simulink library "BechamoNasaOpenModels"  (R2024b)
settings: Solver=VariableStepAuto  StartTime=0.0  StopTime=10.0  RelTol=1e-3
values from neighbouring files (symbols this model uses):
  Cl_aileron_wing_1 = Cl_mat.Claileron_wing.axes1.value    [setupMavrik.m]
  Cl_aileron_wing_2 = Cl_mat.Claileron_wing.axes2.value    [setupMavrik.m]
  Cl_aileron_wing_3 = Cl_mat.Claileron_wing.axes3.value    [setupMavrik.m]
  Cl_aileron_wing_val = Cl_mat.Claileron_wing.value    [setupMavrik.m]
  Cl_elevator_tail_1 = Cl_mat.Clelevator_tail.axes1.value    [setupMavrik.m]
  Cl_elevator_tail_2 = Cl_mat.Clelevator_tail.axes2.value    [setupMavrik.m]
  Cl_elevator_tail_3 = Cl_mat.Clelevator_tail.axes3.value    [setupMavrik.m]
  Cl_elevator_tail_val = Cl_mat.Clelevator_tail.value    [setupMavrik.m]
  Cl_flap_wing_1 = Cl_mat.Clflap_wing.axes1.value    [setupMavrik.m]
  Cl_flap_wing_2 = Cl_mat.Clflap_wing.axes2.value    [setupMavrik.m]
  Cl_flap_wing_3 = Cl_mat.Clflap_wing.axes3.value    [setupMavrik.m]
  Cl_flap_wing_val = Cl_mat.Clflap_wing.value    [setupMavrik.m]
  Cl_hover_fuse_1 = Cl_mat.Clhover_fuse.axes1.value    [setupMavrik.m]
  Cl_hover_fuse_2 = Cl_mat.Clhover_fuse.axes2.value    [setupMavrik.m]
  Cl_hover_fuse_3 = Cl_mat.Clhover_fuse.axes3.value    [setupMavrik.m]
  Cl_hover_fuse_val = Cl_mat.Clhover_fuse.value    [setupMavrik.m]
  Cl_rudder_tail_1 = Cl_mat.Clrudder_tail.axes1.value    [setupMavrik.m]
  Cl_rudder_tail_2 = Cl_mat.Clrudder_tail.axes2.value    [setupMavrik.m]
  Cl_rudder_tail_3 = Cl_mat.Clrudder_tail.axes3.value    [setupMavrik.m]
  Cl_rudder_tail_val = Cl_mat.Clrudder_tail.value    [setupMavrik.m]
  Cl_tail_1 = Cl_mat.Cltail.axes1.value    [setupMavrik.m]
  Cl_tail_2 = Cl_mat.Cltail.axes2.value    [setupMavrik.m]
  Cl_tail_3 = Cl_mat.Cltail.axes3.value    [setupMavrik.m]
  Cl_tail_damp_p_1 = Cl_mat.Cltail_damp_p.axes1.value    [setupMavrik.m]
  Cl_tail_damp_p_2 = Cl_mat.Cltail_damp_p.axes2.value    [setupMavrik.m]
  Cl_tail_damp_p_3 = Cl_mat.Cltail_damp_p.axes3.value    [setupMavrik.m]
  Cl_tail_damp_p_val = Cl_mat.Cltail_damp_p.value    [setupMavrik.m]
  Cl_tail_damp_q_1 = Cl_mat.Cltail_damp_q.axes1.value    [setupMavrik.m]
  Cl_tail_damp_q_2 = Cl_mat.Cltail_damp_q.axes2.value    [setupMavrik.m]
  Cl_tail_damp_q_3 = Cl_mat.Cltail_damp_q.axes3.value    [setupMavrik.m]
  Cl_tail_damp_q_val = Cl_mat.Cltail_damp_q.value    [setupMavrik.m]
  Cl_tail_damp_r_1 = Cl_mat.Cltail_damp_r.axes1.value    [setupMavrik.m]
  Cl_tail_damp_r_2 = Cl_mat.Cltail_damp_r.axes2.value    [setupMavrik.m]
  Cl_tail_damp_r_3 = Cl_mat.Cltail_damp_r.axes3.value    [setupMavrik.m]
  Cl_tail_damp_r_val = Cl_mat.Cltail_damp_r.value    [setupMavrik.m]
  Cl_tail_val = Cl_mat.Cltail.value    [setupMavrik.m]
  Cl_wing_1 = Cl_mat.Clwing.axes1.value    [setupMavrik.m]
  Cl_wing_2 = Cl_mat.Clwing.axes2.value    [setupMavrik.m]
  Cl_wing_3 = Cl_mat.Clwing.axes3.value    [setupMavrik.m]
  Cl_wing_damp_p_1 = Cl_mat.Clwing_damp_p.axes1.value    [setupMavrik.m]
  Cl_wing_damp_p_2 = Cl_mat.Clwing_damp_p.axes2.value    [setupMavrik.m]
  Cl_wing_damp_p_3 = Cl_mat.Clwing_damp_p.axes3.value    [setupMavrik.m]
  Cl_wing_damp_p_val = Cl_mat.Clwing_damp_p.value    [setupMavrik.m]
  Cl_wing_damp_q_1 = Cl_mat.Clwing_damp_q.axes1.value    [setupMavrik.m]
  Cl_wing_damp_q_2 = Cl_mat.Clwing_damp_q.axes2.value    [setupMavrik.m]
  Cl_wing_damp_q_3 = Cl_mat.Clwing_damp_q.axes3.value    [setupMavrik.m]
  Cl_wing_damp_q_val = Cl_mat.Clwing_damp_q.value    [setupMavrik.m]
  Cl_wing_damp_r_1 = Cl_mat.Clwing_damp_r.axes1.value    [setupMavrik.m]
  Cl_wing_damp_r_2 = Cl_mat.Clwing_damp_r.axes2.value    [setupMavrik.m]
  Cl_wing_damp_r_3 = Cl_mat.Clwing_damp_r.axes3.value    [setupMavrik.m]
  Cl_wing_damp_r_val = Cl_mat.Clwing_damp_r.value    [setupMavrik.m]
  Cl_wing_val = Cl_mat.Clwing.value    [setupMavrik.m]
  Cm_aileron_wing_1 = Cm_mat.Cmaileron_wing.axes1.value    [setupMavrik.m]
  Cm_aileron_wing_2 = Cm_mat.Cmaileron_wing.axes2.value    [setupMavrik.m]
  Cm_aileron_wing_3 = Cm_mat.Cmaileron_wing.axes3.value    [setupMavrik.m]
  Cm_aileron_wing_val = Cm_mat.Cmaileron_wing.value    [setupMavrik.m]
  Cm_elevator_tail_1 = Cm_mat.Cmelevator_tail.axes1.value    [setupMavrik.m]
  Cm_elevator_tail_2 = Cm_mat.Cmelevator_tail.axes2.value    [setupMavrik.m]
  Cm_elevator_tail_3 = Cm_mat.Cmelevator_tail.axes3.value    [setupMavrik.m]
  Cm_elevator_tail_val = Cm_mat.Cmelevator_tail.value    [setupMavrik.m]
  Cm_flap_wing_1 = Cm_mat.Cmflap_wing.axes1.value    [setupMavrik.m]
  Cm_flap_wing_2 = Cm_mat.Cmflap_wing.axes2.value    [setupMavrik.m]
  Cm_flap_wing_3 = Cm_mat.Cmflap_wing.axes3.value    [setupMavrik.m]
  Cm_flap_wing_val = Cm_mat.Cmflap_wing.value    [setupMavrik.m]
  Cm_hover_fuse_1 = Cm_mat.Cmhover_fuse.axes1.value    [setupMavrik.m]
  Cm_hover_fuse_2 = Cm_mat.Cmhover_fuse.axes2.value    [setupMavrik.m]
  Cm_hover_fuse_3 = Cm_mat.Cmhover_fuse.axes3.value    [setupMavrik.m]
  Cm_hover_fuse_val = Cm_mat.Cmhover_fuse.value    [setupMavrik.m]
  Cm_rudder_tail_1 = Cm_mat.Cmrudder_tail.axes1.value    [setupMavrik.m]
  Cm_rudder_tail_2 = Cm_mat.Cmrudder_tail.axes2.value    [setupMavrik.m]
  Cm_rudder_tail_3 = Cm_mat.Cmrudder_tail.axes3.value    [setupMavrik.m]
  Cm_rudder_tail_val = Cm_mat.Cmrudder_tail.value    [setupMavrik.m]
  Cm_tail_1 = Cm_mat.Cmtail.axes1.value    [setupMavrik.m]
  Cm_tail_2 = Cm_mat.Cmtail.axes2.value    [setupMavrik.m]
  Cm_tail_3 = Cm_mat.Cmtail.axes3.value    [setupMavrik.m]
  Cm_tail_damp_p_1 = Cm_mat.Cmtail_damp_p.axes1.value    [setupMavrik.m]
  Cm_tail_damp_p_2 = Cm_mat.Cmtail_damp_p.axes2.value    [setupMavrik.m]
  Cm_tail_damp_p_3 = Cm_mat.Cmtail_damp_p.axes3.value    [setupMavrik.m]
  Cm_tail_damp_p_val = Cm_mat.Cmtail_damp_p.value    [setupMavrik.m]
  Cm_tail_damp_q_1 = Cm_mat.Cmtail_damp_q.axes1.value    [setupMavrik.m]
  Cm_tail_damp_q_2 = Cm_mat.Cmtail_damp_q.axes2.value    [setupMavrik.m]
  Cm_tail_damp_q_3 = Cm_mat.Cmtail_damp_q.axes3.value    [setupMavrik.m]
  Cm_tail_damp_q_val = Cm_mat.Cmtail_damp_q.value    [setupMavrik.m]
  Cm_tail_damp_r_1 = Cm_mat.Cmtail_damp_r.axes1.value    [setupMavrik.m]
  Cm_tail_damp_r_2 = Cm_mat.Cmtail_damp_r.axes2.value    [setupMavrik.m]
  Cm_tail_damp_r_3 = Cm_mat.Cmtail_damp_r.axes3.value    [setupMavrik.m]
  Cm_tail_damp_r_val = Cm_mat.Cmtail_damp_r.value    [setupMavrik.m]
  Cm_tail_val = Cm_mat.Cmtail.value    [setupMavrik.m]
  Cm_wing_1 = Cm_mat.Cmwing.axes1.value    [setupMavrik.m]
  Cm_wing_2 = Cm_mat.Cmwing.axes2.value    [setupMavrik.m]
  Cm_wing_3 = Cm_mat.Cmwing.axes3.value    [setupMavrik.m]
  Cm_wing_damp_p_1 = Cm_mat.Cmwing_damp_p.axes1.value    [setupMavrik.m]
  Cm_wing_damp_p_2 = Cm_mat.Cmwing_damp_p.axes2.value    [setupMavrik.m]
  Cm_wing_damp_p_3 = Cm_mat.Cmwing_damp_p.axes3.value    [setupMavrik.m]
  Cm_wing_damp_p_val = Cm_mat.Cmwing_damp_p.value    [setupMavrik.m]
  Cm_wing_damp_q_1 = Cm_mat.Cmwing_damp_q.axes1.value    [setupMavrik.m]
  Cm_wing_damp_q_2 = Cm_mat.Cmwing_damp_q.axes2.value    [setupMavrik.m]
  Cm_wing_damp_q_3 = Cm_mat.Cmwing_damp_q.axes3.value    [setupMavrik.m]
  Cm_wing_damp_q_val = Cm_mat.Cmwing_damp_q.value    [setupMavrik.m]
  Cm_wing_damp_r_1 = Cm_mat.Cmwing_damp_r.axes1.value    [setupMavrik.m]
  Cm_wing_damp_r_2 = Cm_mat.Cmwing_damp_r.axes2.value    [setupMavrik.m]
  Cm_wing_damp_r_3 = Cm_mat.Cmwing_damp_r.axes3.value    [setupMavrik.m]
  Cm_wing_damp_r_val = Cm_mat.Cmwing_damp_r.value    [setupMavrik.m]
  Cm_wing_val = Cm_mat.Cmwing.value    [setupMavrik.m]
  Cn_aileron_wing_1 = Cn_mat.Cnaileron_wing.axes1.value    [setupMavrik.m]
  Cn_aileron_wing_2 = Cn_mat.Cnaileron_wing.axes2.value    [setupMavrik.m]
  Cn_aileron_wing_3 = Cn_mat.Cnaileron_wing.axes3.value    [setupMavrik.m]
  Cn_aileron_wing_val = Cn_mat.Cnaileron_wing.value    [setupMavrik.m]
  Cn_elevator_tail_1 = Cn_mat.Cnelevator_tail.axes1.value    [setupMavrik.m]
  Cn_elevator_tail_2 = Cn_mat.Cnelevator_tail.axes2.value    [setupMavrik.m]
  Cn_elevator_tail_3 = Cn_mat.Cnelevator_tail.axes3.value    [setupMavrik.m]
  Cn_elevator_tail_val = Cn_mat.Cnelevator_tail.value    [setupMavrik.m]
  Cn_flap_wing_1 = Cn_mat.Cnflap_wing.axes1.value    [setupMavrik.m]
  Cn_flap_wing_2 = Cn_mat.Cnflap_wing.axes2.value    [setupMavrik.m]
  Cn_flap_wing_3 = Cn_mat.Cnflap_wing.axes3.value    [setupMavrik.m]
  Cn_flap_wing_val = Cn_mat.Cnflap_wing.value    [setupMavrik.m]
  Cn_hover_fuse_1 = Cn_mat.Cnhover_fuse.axes1.value    [setupMavrik.m]
  Cn_hover_fuse_2 = Cn_mat.Cnhover_fuse.axes2.value    [setupMavrik.m]
  Cn_hover_fuse_3 = Cn_mat.Cnhover_fuse.axes3.value    [setupMavrik.m]
  Cn_hover_fuse_val = Cn_mat.Cnhover_fuse.value    [setupMavrik.m]
  ... (+319 more)
libraries: matrix_library x15, sharedtransform x2, $bdroot x1, shared6dof x1
(part 1 of 19)
settings Model: Creator=MichaelPiedmonte  LastModifiedBy=DivyangAmin

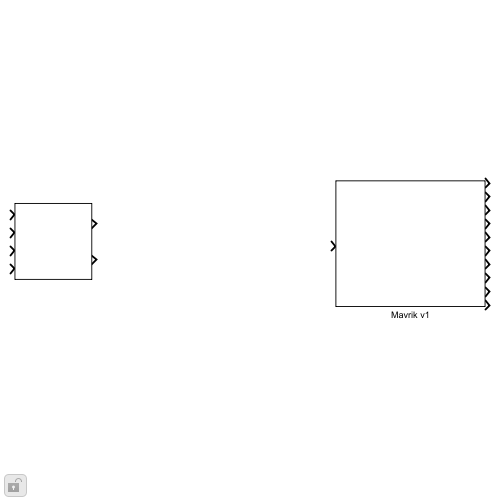
[thumbnail: Simulink's stored preview of the top-level diagram]
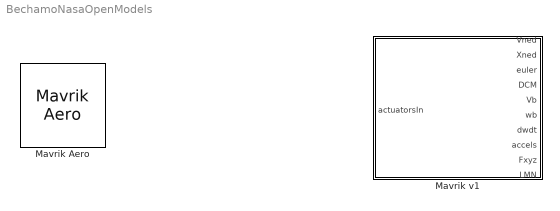
== system BechamoNasaOpenModels ==
  Mavrik Aero : $bdroot/Mavrik v1/Mavrik Aero  SystemSampleTime=-1  VariantActivationTime=update diagram  AllowFlexibleInterface=on  Latency=0  AutoFrameSizeCalculation=off
  Mavrik v1 : Subsystem  mask{uvw_init=0, pqr_init=0, euler_init=0, xyz_init=0, mass=0, inertia=0}
      mask prompts: uvw_init "uvw initial values"; pqr_init "pqr initial values"; euler_init "euler angle initial values"; xyz_init "xyz initial values"; mass "Mass (kg)"; inertia "Inertia (kg m^2)"

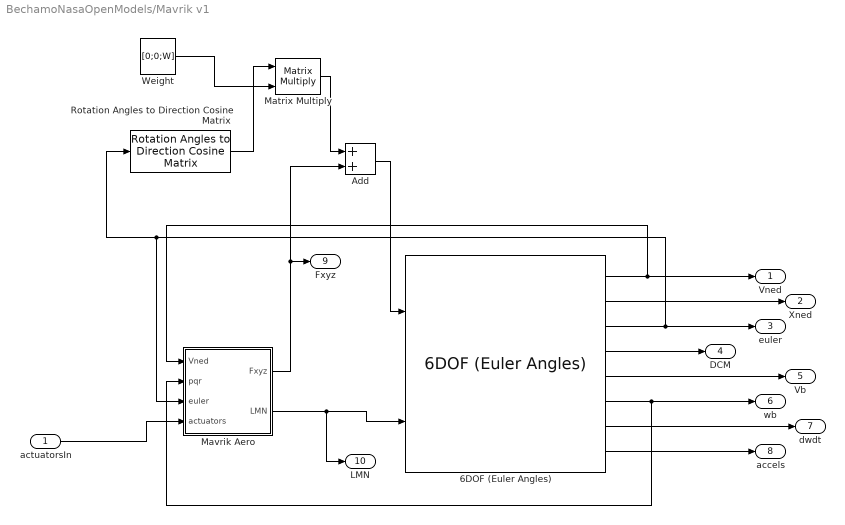
== system BechamoNasaOpenModels/Mavrik v1 ==
  actuatorsIn : Inport
  6DOF (Euler Angles) : shared6dof/6DOF (Euler Angles)  units=Metric (MKS)  mtype=Fixed  rep=Euler Angles  xme_0=xyz_init  Vm_0=uvw_init  eul_0=euler_init  pm_0=pqr_init  mass_0=mass  mass_e=0.5  mass_f=2.0  inertia=inertia  inertia_e=eye(3)  inertia_f=2*eye(3)  k_quat=1.0  vre_flag=on  abi_flag=off  aMode=0  xme_statename=''  Vm_statename=''  eul_statename=''  quat_statename=''  pm_statename=''  mass_statename=''
  Add : Sum
  Matrix Multiply : Product  Multiplication=Matrix(*)
  Mavrik Aero : Subsystem
  Rotation Angles to Direction Cosine Matrix : sharedtransform/Rotation Angles to Direction Cosine Matrix  rotationOrder=ZYX  aMode=aMode
  Weight : Constant  Value=[0;0;W]
  Vned : Outport
  Xned : Outport  Port=2
  euler : Outport  Port=3
  DCM : Outport  Port=4
  Vb : Outport  Port=5
  wb : Outport  Port=6
  dwdt : Outport  Port=7
  accels : Outport  Port=8
  Fxyz : Outport  Port=9
  LMN : Outport  Port=10
  wires:
  Mavrik Aero/2(LMN) -> LMN/1, 6DOF (Euler Angles)/2
  6DOF (Euler Angles)/6 -> Mavrik Aero/2(pqr), wb/1
  actuatorsIn/1 -> Mavrik Aero/4(actuators)
  Mavrik Aero/1(Fxyz) -> Add/2, Fxyz/1
  6DOF (Euler Angles)/1 -> Mavrik Aero/1(Vned), Vned/1
  6DOF (Euler Angles)/2 -> Xned/1
  6DOF (Euler Angles)/5 -> Vb/1
  6DOF (Euler Angles)/3 -> Rotation Angles to Direction Cosine Matrix/1, Mavrik Aero/3(euler), euler/1
  6DOF (Euler Angles)/4 -> DCM/1
  6DOF (Euler Angles)/7 -> dwdt/1
  6DOF (Euler Angles)/8 -> accels/1
  Add/1 -> 6DOF (Euler Angles)/1
  Matrix Multiply/1 -> Add/1
  Rotation Angles to Direction Cosine Matrix/1 -> Matrix Multiply/1
  Weight/1 -> Matrix Multiply/2

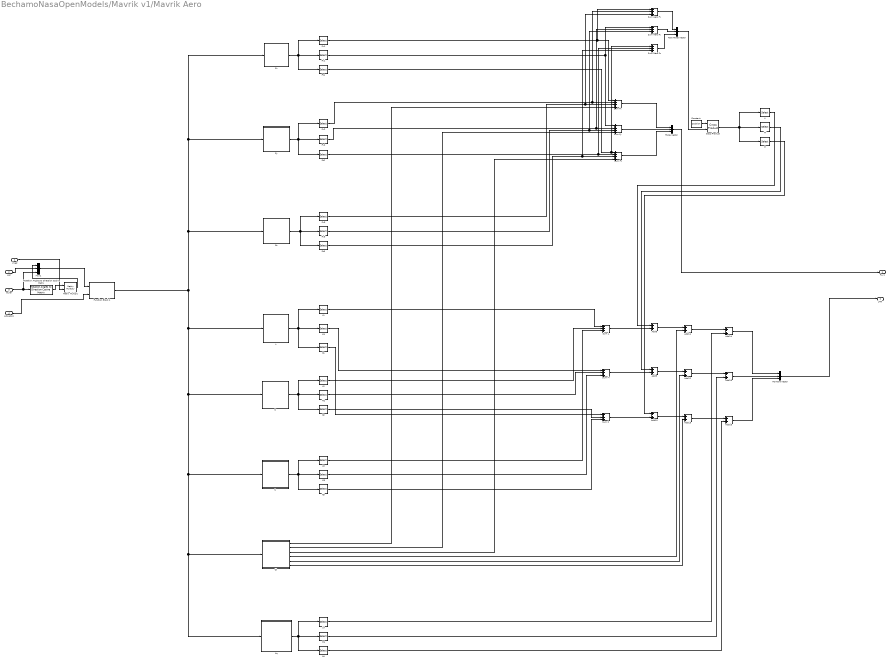
== system BechamoNasaOpenModels/Mavrik v1/Mavrik Aero ==
  Vned : Inport
  pqr : Inport  Port=2
  euler : Inport  Port=3
  actuators : Inport  Port=4
  Add{8..16} (9 alike) : Sum
  Aero Force Vector : Mux  Inputs=3
  Constant : Constant  Value=position
  Cross Product : matrix_library/Cross Product
  Ct : Subsystem
  Cx : Subsystem
  Cy : Subsystem
  Cz : Subsystem
  Force Vector : Mux  Inputs=3
  Function Block 1 : MATLAB Function  TreatAsAtomicUnit=on
  Fx1 : Selector  InputPortWidth=3  IndexOptions=Starting index (dialog)  Indices=[1]  OutputSizes=1
  Fx2 : Selector  InputPortWidth=3  IndexOptions=Starting index (dialog)  Indices=[1]  OutputSizes=1
  Fx3 : Selector  InputPortWidth=3  IndexOptions=Starting index (dialog)  Indices=[1]  OutputSizes=1
  Fy1 : Selector  InputPortWidth=3  IndexOptions=Starting index (dialog)  Indices=[2]  OutputSizes=1
  Fy2 : Selector  InputPortWidth=3  IndexOptions=Starting index (dialog)  Indices=[2]  OutputSizes=1
  Fy3 : Selector  InputPortWidth=3  IndexOptions=Starting index (dialog)  Indices=[2]  OutputSizes=1
  Fz1 : Selector  InputPortWidth=3  IndexOptions=Starting index (dialog)  Indices=[3]  OutputSizes=1
  Fz2 : Selector  InputPortWidth=3  IndexOptions=Starting index (dialog)  Indices=[3]  OutputSizes=1
  Fz3 : Selector  InputPortWidth=3  IndexOptions=Starting index (dialog)  Indices=[3]  OutputSizes=1
  Kq : Subsystem
  L : Subsystem
  L' : Selector  InputPortWidth=3  IndexOptions=Starting index (dialog)  Indices=[1]  OutputSizes=1
  L{1..4} (4 alike) : Selector  InputPortWidth=3  IndexOptions=Starting index (dialog)  Indices=[1]  OutputSizes=1
  M : Subsystem
  M' : Selector  InputPortWidth=3  IndexOptions=Starting index (dialog)  Indices=[2]  OutputSizes=1
  M{1..4} (4 alike) : Selector  InputPortWidth=3  IndexOptions=Starting index (dialog)  Indices=[2]  OutputSizes=1
  Matrix Multiply : Product  Multiplication=Matrix(*)
  Moment Vector : Mux  Inputs=3
  Mux1 : Mux  Inputs=3
  N : Subsystem
  N' : Selector  InputPortWidth=3  IndexOptions=Starting index (dialog)  Indices=[3]  OutputSizes=1
  N{1..4} (4 alike) : Selector  InputPortWidth=3  IndexOptions=Starting index (dialog)  Indices=[3]  OutputSizes=1
  Rotation Angles to Direction Cosine Matrix : sharedtransform/Rotation Angles to Direction Cosine Matrix  rotationOrder=ZYX  aMode=aMode
  Sum Aero Fx : Sum  Inputs=+++
  Sum Aero Fy : Sum  Inputs=+++
  Sum Aero Fz : Sum  Inputs=+++
  Sum Fx : Sum  Inputs=++++
  Sum Fy : Sum  Inputs=++++
  Sum Fz : Sum  Inputs=++++
  Sum L : Sum  Inputs=+++
  Sum M : Sum  Inputs=+++
  Sum N : Sum  Inputs=+++
  Fxyz : Outport
  LMN : Outport  Port=2
  wires:
  Fz1/1 -> Sum Aero Fz/1, Sum Fz/1
  Function Block 1/1(y) -> Cz/1(u), Cx/1(u), Cy/1(u), L/1(u), Kq/1(u), Ct/1(u19), N/1(u), M/1(u)
  Ct/6(Out6) -> Add13/2
  L2/1 -> Sum L/2
  Fz3/1 -> Sum Aero Fz/3, Sum Fz/3
  N1/1 -> Sum N/1
  Fx1/1 -> Sum Aero Fx/1, Sum Fx/1
  Add8/1 -> Add11/1
  Kq/1(Out1) -> L4/1, N4/1, M4/1
  Sum N/1 -> Add10/2
  Ct/5(Out5) -> Add12/2
  Force Vector/1 -> Fxyz/1
  Ct/3(Out3) -> Sum Fz/4
  Sum L/1 -> Add8/2
  Sum Fy/1 -> Force Vector/2
  Fx2/1 -> Sum Aero Fx/2, Sum Fx/2
  euler/1 -> Mux1/3, Rotation Angles to Direction Cosine Matrix/1
  L3/1 -> Sum L/3
  N/1(Out1) -> L3/1, N3/1, M3/1
  Fy1/1 -> Sum Fy/1, Sum Aero Fy/1
  L'/1 -> Add8/1
  Fz2/1 -> Sum Aero Fz/2, Sum Fz/2
  Cz/1(Out1) -> Fz3/1, Fx3/1, Fy3/1
  Add9/1 -> Add12/1
  M4/1 -> Add15/2
  Sum Fx/1 -> Force Vector/1
  N'/1 -> Add10/1
  Add15/1 -> Moment Vector/2
  pqr/1 -> Mux1/2
  Ct/1(Out1) -> Sum Fx/4
  L/1(Out1) -> M1/1, L1/1, N1/1
  M3/1 -> Sum M/3
  Sum M/1 -> Add9/2
  Fy2/1 -> Sum Aero Fy/2, Sum Fy/2
  M/1(Out1) -> L2/1, N2/1, M2/1
  Add14/1 -> Moment Vector/1
  Fx3/1 -> Sum Aero Fx/3, Sum Fx/3
  Add11/1 -> Add14/1
  Add12/1 -> Add15/1
  Rotation Angles to Direction Cosine Matrix/1 -> Matrix Multiply/1
  Add16/1 -> Moment Vector/3
  Cx/1(Out1) -> Fz1/1, Fx1/1, Fy1/1
  N2/1 -> Sum N/2
  Cy/1(Out1) -> Fy2/1, Fx2/1, Fz2/1
  Add10/1 -> Add13/1
  Matrix Multiply/1 -> Mux1/1  "uvw"
  Cross Product/1 -> L'/1, M'/1, N'/1
  Ct/4(Out4) -> Add11/2
  M'/1 -> Add9/1
  Ct/2(Out2) -> Sum Fy/4
  M1/1 -> Sum M/1
  Mux1/1 -> Function Block 1/1(u)
  L4/1 -> Add14/2
  L1/1 -> Sum L/1
  N3/1 -> Sum N/3
  Fy3/1 -> Sum Aero Fy/3, Sum Fy/3
  Sum Fz/1 -> Force Vector/3
  Constant/1 -> Cross Product/1
  M2/1 -> Sum M/2
  actuators/1 -> Function Block 1/2(actuators)
  Add13/1 -> Add16/1
  N4/1 -> Add16/2
  Vned/1 -> Matrix Multiply/2
  Moment Vector/1 -> LMN/1
  Sum Aero Fz/1 -> Aero Force Vector/3
  Sum Aero Fy/1 -> Aero Force Vector/2
  Sum Aero Fx/1 -> Aero Force Vector/1
  Aero Force Vector/1 -> Cross Product/2

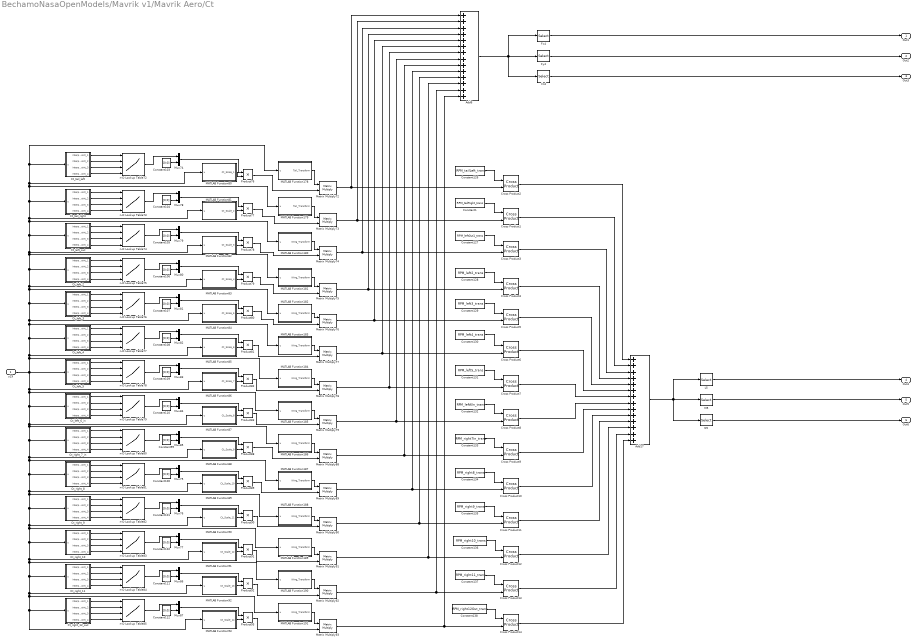
== system BechamoNasaOpenModels/Mavrik v1/Mavrik Aero/Ct ==
  u19 : Inport
  Add17 : Sum  Inputs=++++++++++++++
  Add6 : Sum  Inputs=++++++++++++++
  Constant1 : Constant  Value=RPM_tailRight_trans
  Constant{99..112} (14 alike) : Constant  Value=[0;0]
  Constant126 : Constant  Value=RPM_tailLeft_trans
  Constant127 : Constant  Value=RPM_leftOut1_trans
  Constant128 : Constant  Value=RPM_left2_trans
  Constant129 : Constant  Value=RPM_left3_trans
  Constant130 : Constant  Value=RPM_left4_trans
  Constant131 : Constant  Value=RPM_left5_trans
  Constant132 : Constant  Value=RPM_left6In_trans
  Constant133 : Constant  Value=RPM_right7In_trans
  Constant134 : Constant  Value=RPM_right8_trans
  Constant135 : Constant  Value=RPM_right9_trans
  Constant136 : Constant  Value=RPM_right10_trans
  Constant137 : Constant  Value=RPM_right11_trans
  Constant138 : Constant  Value=RPM_right12Out_trans
  Cross Product{1..14} (14 alike) : matrix_library/Cross Product
  Ct_left_2 : MATLAB Function  TreatAsAtomicUnit=on
  Ct_left_3 : MATLAB Function  TreatAsAtomicUnit=on
  Ct_left_4 : MATLAB Function  TreatAsAtomicUnit=on
  Ct_left_5 : MATLAB Function  TreatAsAtomicUnit=on
  Ct_left_6_in : MATLAB Function  TreatAsAtomicUnit=on
  Ct_left_out : MATLAB Function  TreatAsAtomicUnit=on
  Ct_right_10 : MATLAB Function  TreatAsAtomicUnit=on
  Ct_right_11 : MATLAB Function  TreatAsAtomicUnit=on
  Ct_right_12_out : MATLAB Function  TreatAsAtomicUnit=on
  Ct_right_7_in : MATLAB Function  TreatAsAtomicUnit=on
  Ct_right_8 : MATLAB Function  TreatAsAtomicUnit=on
  Ct_right_9 : MATLAB Function  TreatAsAtomicUnit=on
  Ct_tail_left : MATLAB Function  TreatAsAtomicUnit=on
  Ct_tail_right : MATLAB Function  TreatAsAtomicUnit=on
  Fx4 : Selector  InputPortWidth=3  IndexOptions=Starting index (dialog)  Indices=[1]  OutputSizes=1
  Fy4 : Selector  InputPortWidth=3  IndexOptions=Starting index (dialog)  Indices=[2]  OutputSizes=1
  Fz4 : Selector  InputPortWidth=3  IndexOptions=Starting index (dialog)  Indices=[3]  OutputSizes=1
  L5 : Selector  InputPortWidth=3  IndexOptions=Starting index (dialog)  Indices=[1]  OutputSizes=1
  M5 : Selector  InputPortWidth=3  IndexOptions=Starting index (dialog)  Indices=[2]  OutputSizes=1
  MATLAB Function178 : MATLAB Function  TreatAsAtomicUnit=on
  MATLAB Function179 : MATLAB Function  TreatAsAtomicUnit=on
  MATLAB Function180 : MATLAB Function  TreatAsAtomicUnit=on
  MATLAB Function181 : MATLAB Function  TreatAsAtomicUnit=on
  MATLAB Function182 : MATLAB Function  TreatAsAtomicUnit=on
  MATLAB Function183 : MATLAB Function  TreatAsAtomicUnit=on
  MATLAB Function184 : MATLAB Function  TreatAsAtomicUnit=on
  MATLAB Function185 : MATLAB Function  TreatAsAtomicUnit=on
  MATLAB Function186 : MATLAB Function  TreatAsAtomicUnit=on
  MATLAB Function187 : MATLAB Function  TreatAsAtomicUnit=on
  MATLAB Function188 : MATLAB Function  TreatAsAtomicUnit=on
  MATLAB Function189 : MATLAB Function  TreatAsAtomicUnit=on
  MATLAB Function190 : MATLAB Function  TreatAsAtomicUnit=on
  MATLAB Function191 : MATLAB Function  TreatAsAtomicUnit=on
  MATLAB Function80 : MATLAB Function  TreatAsAtomicUnit=on
  MATLAB Function81 : MATLAB Function  TreatAsAtomicUnit=on
  MATLAB Function82 : MATLAB Function  TreatAsAtomicUnit=on
  MATLAB Function83 : MATLAB Function  TreatAsAtomicUnit=on
  MATLAB Function84 : MATLAB Function  TreatAsAtomicUnit=on
  MATLAB Function85 : MATLAB Function  TreatAsAtomicUnit=on
  MATLAB Function86 : MATLAB Function  TreatAsAtomicUnit=on
  MATLAB Function87 : MATLAB Function  TreatAsAtomicUnit=on
  MATLAB Function88 : MATLAB Function  TreatAsAtomicUnit=on
  MATLAB Function89 : MATLAB Function  TreatAsAtomicUnit=on
  MATLAB Function90 : MATLAB Function  TreatAsAtomicUnit=on
  MATLAB Function91 : MATLAB Function  TreatAsAtomicUnit=on
  MATLAB Function92 : MATLAB Function  TreatAsAtomicUnit=on
  MATLAB Function93 : MATLAB Function  TreatAsAtomicUnit=on
  Matrix Multiply{72..79,88..93} (14 alike) : Product  Multiplication=Matrix(*)
  Mux{74..87} (14 alike) : Mux  Inputs=2
  N5 : Selector  InputPortWidth=3  IndexOptions=Starting index (dialog)  Indices=[3]  OutputSizes=1
  Product{76..83,88..93} (14 alike) : Product
  n-D Lookup Table72 : Lookup_n-D  NumberOfTableDimensions=4  BreakpointsForDimension1=Ct_tail_left_1  BreakpointsForDimension2=Ct_tail_left_2  BreakpointsForDimension3=Ct_tail_left_3  BreakpointsForDimension4=Ct_tail_left_4  BreakpointsForDimension5=Cn_wing_damp_r_5  BreakpointsForDimension6=Cn_wing_damp_r_6  BreakpointsForDimension7=CX_flap_wing_7  Table=Ct_tail_left_val  InternalRulePriority=Speed  OutDataTypeStr=Inherit: Inherit via back propagation  RndMeth=Simplest
      settings: InputPortMap=u0,u1,u2,u3
  n-D Lookup Table73 : Lookup_n-D  NumberOfTableDimensions=4  BreakpointsForDimension1=Ct_tail_right_1  BreakpointsForDimension2=Ct_tail_right_2  BreakpointsForDimension3=Ct_tail_right_3  BreakpointsForDimension4=Ct_tail_right_4  BreakpointsForDimension5=Cn_wing_damp_r_5  BreakpointsForDimension6=Cn_wing_damp_r_6  BreakpointsForDimension7=CX_flap_wing_7  Table=Ct_tail_right_val  InternalRulePriority=Speed  OutDataTypeStr=Inherit: Inherit via back propagation  RndMeth=Simplest
      settings: InputPortMap=u0,u1,u2,u3
  n-D Lookup Table74 : Lookup_n-D  NumberOfTableDimensions=4  BreakpointsForDimension1=Ct_left_out_1  BreakpointsForDimension2=Ct_left_out_2  BreakpointsForDimension3=Ct_left_out_3  BreakpointsForDimension4=Ct_left_out_4  BreakpointsForDimension5=Cn_wing_damp_r_5  BreakpointsForDimension6=Cn_wing_damp_r_6  BreakpointsForDimension7=CX_flap_wing_7  Table=Ct_left_out_val  InternalRulePriority=Speed  OutDataTypeStr=Inherit: Inherit via back propagation  RndMeth=Simplest
      settings: InputPortMap=u0,u1,u2,u3
  n-D Lookup Table75 : Lookup_n-D  NumberOfTableDimensions=4  BreakpointsForDimension1=Ct_left_2_1  BreakpointsForDimension2=Ct_left_2_2  BreakpointsForDimension3=Ct_left_2_3  BreakpointsForDimension4=Ct_left_2_4  BreakpointsForDimension5=Cn_wing_damp_r_5  BreakpointsForDimension6=Cn_wing_damp_r_6  BreakpointsForDimension7=CX_flap_wing_7  Table=Ct_left_2_val  InternalRulePriority=Speed  OutDataTypeStr=Inherit: Inherit via back propagation  RndMeth=Simplest
      settings: InputPortMap=u0,u1,u2,u3
  n-D Lookup Table76 : Lookup_n-D  NumberOfTableDimensions=4  BreakpointsForDimension1=Ct_left_3_1  BreakpointsForDimension2=Ct_left_3_2  BreakpointsForDimension3=Ct_left_3_3  BreakpointsForDimension4=Ct_left_3_4  BreakpointsForDimension5=Cn_wing_damp_r_5  BreakpointsForDimension6=Cn_wing_damp_r_6  BreakpointsForDimension7=CX_flap_wing_7  Table=Ct_left_3_val  InternalRulePriority=Speed  OutDataTypeStr=Inherit: Inherit via back propagation  RndMeth=Simplest
      settings: InputPortMap=u0,u1,u2,u3
  n-D Lookup Table77 : Lookup_n-D  NumberOfTableDimensions=4  BreakpointsForDimension1=Ct_left_4_1  BreakpointsForDimension2=Ct_left_4_2  BreakpointsForDimension3=Ct_left_4_3  BreakpointsForDimension4=Ct_left_4_4  BreakpointsForDimension5=Cn_wing_damp_r_5  BreakpointsForDimension6=Cn_wing_damp_r_6  BreakpointsForDimension7=CX_flap_wing_7  Table=Ct_left_4_val  InternalRulePriority=Speed  OutDataTypeStr=Inherit: Inherit via back propagation  RndMeth=Simplest
      settings: InputPortMap=u0,u1,u2,u3
  n-D Lookup Table78 : Lookup_n-D  NumberOfTableDimensions=4  BreakpointsForDimension1=Ct_left_5_1  BreakpointsForDimension2=Ct_left_5_2  BreakpointsForDimension3=Ct_left_5_3  BreakpointsForDimension4=Ct_left_5_4  BreakpointsForDimension5=Cn_wing_damp_r_5  BreakpointsForDimension6=Cn_wing_damp_r_6  BreakpointsForDimension7=CX_flap_wing_7  Table=Ct_left_5_val  InternalRulePriority=Speed  OutDataTypeStr=Inherit: Inherit via back propagation  RndMeth=Simplest
      settings: InputPortMap=u0,u1,u2,u3
  n-D Lookup Table79 : Lookup_n-D  NumberOfTableDimensions=4  BreakpointsForDimension1=Ct_left_6_in_1  BreakpointsForDimension2=Ct_left_6_in_2  BreakpointsForDimension3=Ct_left_6_in_3  BreakpointsForDimension4=Ct_left_6_in_4  BreakpointsForDimension5=Cn_wing_damp_r_5  BreakpointsForDimension6=Cn_wing_damp_r_6  BreakpointsForDimension7=CX_flap_wing_7  Table=Ct_left_6_in_val  InternalRulePriority=Speed  OutDataTypeStr=Inherit: Inherit via back propagation  RndMeth=Simplest
      settings: InputPortMap=u0,u1,u2,u3
  n-D Lookup Table80 : Lookup_n-D  NumberOfTableDimensions=4  BreakpointsForDimension1=Ct_right_7_in_1  BreakpointsForDimension2=Ct_right_7_in_2  BreakpointsForDimension3=Ct_right_7_in_3  BreakpointsForDimension4=Ct_right_7_in_4  BreakpointsForDimension5=Cn_wing_damp_r_5  BreakpointsForDimension6=Cn_wing_damp_r_6  BreakpointsForDimension7=CX_flap_wing_7  Table=Ct_right_7_in_val  InternalRulePriority=Speed  OutDataTypeStr=Inherit: Inherit via back propagation  RndMeth=Simplest
      settings: InputPortMap=u0,u1,u2,u3
  n-D Lookup Table81 : Lookup_n-D  NumberOfTableDimensions=4  BreakpointsForDimension1=Ct_right_8_1  BreakpointsForDimension2=Ct_right_8_2  BreakpointsForDimension3=Ct_right_8_3  BreakpointsForDimension4=Ct_right_8_4  BreakpointsForDimension5=Cn_wing_damp_r_5  BreakpointsForDimension6=Cn_wing_damp_r_6  BreakpointsForDimension7=CX_flap_wing_7  Table=Ct_right_8_val  InternalRulePriority=Speed  OutDataTypeStr=Inherit: Inherit via back propagation  RndMeth=Simplest
      settings: InputPortMap=u0,u1,u2,u3
  n-D Lookup Table82 : Lookup_n-D  NumberOfTableDimensions=4  BreakpointsForDimension1=Ct_right_9_1  BreakpointsForDimension2=Ct_right_9_2  BreakpointsForDimension3=Ct_right_9_3  BreakpointsForDimension4=Ct_right_9_4  BreakpointsForDimension5=Cn_wing_damp_r_5  BreakpointsForDimension6=Cn_wing_damp_r_6  BreakpointsForDimension7=CX_flap_wing_7  Table=Ct_right_9_val  InternalRulePriority=Speed  OutDataTypeStr=Inherit: Inherit via back propagation  RndMeth=Simplest
      settings: InputPortMap=u0,u1,u2,u3
  n-D Lookup Table83 : Lookup_n-D  NumberOfTableDimensions=4  BreakpointsForDimension1=Ct_right_10_1  BreakpointsForDimension2=Ct_right_10_2  BreakpointsForDimension3=Ct_right_10_3  BreakpointsForDimension4=Ct_right_10_4  BreakpointsForDimension5=Cn_wing_damp_r_5  BreakpointsForDimension6=Cn_wing_damp_r_6  BreakpointsForDimension7=CX_flap_wing_7  Table=Ct_right_10_val  InternalRulePriority=Speed  OutDataTypeStr=Inherit: Inherit via back propagation  RndMeth=Simplest
      settings: InputPortMap=u0,u1,u2,u3
  n-D Lookup Table84 : Lookup_n-D  NumberOfTableDimensions=4  BreakpointsForDimension1=Ct_right_11_1  BreakpointsForDimension2=Ct_right_11_2  BreakpointsForDimension3=Ct_right_11_3  BreakpointsForDimension4=Ct_right_11_4  BreakpointsForDimension5=Cn_wing_damp_r_5  BreakpointsForDimension6=Cn_wing_damp_r_6  BreakpointsForDimension7=CX_flap_wing_7  Table=Ct_right_11_val  InternalRulePriority=Speed  OutDataTypeStr=Inherit: Inherit via back propagation  RndMeth=Simplest
      settings: InputPortMap=u0,u1,u2,u3
  n-D Lookup Table85 : Lookup_n-D  NumberOfTableDimensions=4  BreakpointsForDimension1=Ct_right_12_out_1  BreakpointsForDimension2=Ct_right_12_out_2  BreakpointsForDimension3=Ct_right_12_out_3  BreakpointsForDimension4=Ct_right_12_out_4  BreakpointsForDimension5=Cn_wing_damp_r_5  BreakpointsForDimension6=Cn_wing_damp_r_6  BreakpointsForDimension7=CX_flap_wing_7  Table=Ct_right_12_out_val  InternalRulePriority=Speed  OutDataTypeStr=Inherit: Inherit via back propagation  RndMeth=Simplest
      settings: InputPortMap=u0,u1,u2,u3
  Out1 : Outport
  Out2 : Outport  Port=2
  Out3 : Outport  Port=3
  Out4 : Outport  Port=4
  Out5 : Outport  Port=5
  Out6 : Outport  Port=6
  wires:
  Mux85/1 -> Product88/1
  Mux74/1 -> Product76/1
  Mux83/1 -> Product82/1
  n-D Lookup Table78/1 -> Mux83/1
  Cross Product7/1 -> Add17/7
  Mux80/1 -> Product79/1
  Add6/1 -> Fz4/1, Fy4/1, Fx4/1
  Constant127/1 -> Cross Product3/1
  Mux82/1 -> Product81/1
  n-D Lookup Table77/1 -> Mux82/1
  Product83/1 -> Matrix Multiply79/2
  MATLAB Function80/1(Ct_Scale_1) -> Product76/2
  Ct_right_10/4(interp_point_4) -> n-D Lookup Table83/4
  n-D Lookup Table73/1 -> Mux78/1
  Ct_right_10/2(interp_point_2) -> n-D Lookup Table83/2
  Constant109/1 -> Mux83/2
  MATLAB Function183/1(Wing_Transform) -> Matrix Multiply77/1
  Ct_right_10/3(interp_point_3) -> n-D Lookup Table83/3
  MATLAB Function90/1(Ct_Scale_11) -> Product90/2
  Matrix Multiply75/1 -> Add6/4, Cross Product4/2
  Product89/1 -> Matrix Multiply89/2
  Product90/1 -> Matrix Multiply90/2
  Mux76/1 -> Product90/1
  Cross Product5/1 -> Add17/5
  Matrix Multiply90/1 -> Add6/11, Cross Product11/2
  MATLAB Function89/1(Ct_Scale_10) -> Product89/2
  Ct_right_12_out/3(interp_point_3) -> n-D Lookup Table85/3
  n-D Lookup Table80/1 -> Mux85/1
  Product76/1 -> Matrix Multiply72/2
  Mux77/1 -> Product91/1
  Ct_left_out/1(interp_point_1) -> n-D Lookup Table74/1
  Product93/1 -> Matrix Multiply93/2
  Ct_tail_left/1(interp_point_1) -> n-D Lookup Table72/1
  n-D Lookup Table79/1 -> Mux84/1
  Constant130/1 -> Cross Product6/1
  Ct_tail_left/2(interp_point_2) -> n-D Lookup Table72/2
  Add17/1 -> N5/1, L5/1, M5/1
  Ct_left_out/4(interp_point_4) -> n-D Lookup Table74/4
  MATLAB Function91/1(Ct_Scale_12) -> Product91/2
  Constant108/1 -> Mux82/2
  MATLAB Function86/1(Ct_Scale_7) -> Product82/2
  Ct_right_10/1(interp_point_1) -> n-D Lookup Table83/1
  Product88/1 -> Matrix Multiply88/2
  Ct_right_9/1(interp_point_1) -> n-D Lookup Table82/1
  Constant112/1 -> Mux87/2
  Ct_right_8/4(interp_point_4) -> n-D Lookup Table81/4
  Constant134/1 -> Cross Product10/1
  Matrix Multiply91/1 -> Add6/12, Cross Product12/2
  MATLAB Function83/1(Ct_Scale_4) -> Product79/2
  Constant135/1 -> Cross Product11/1
  Product82/1 -> Matrix Multiply78/2
  Constant132/1 -> Cross Product8/1
  Constant102/1 -> Mux77/2
  Matrix Multiply89/1 -> Add6/10, Cross Product10/2
  N5/1 -> Out6/1
  Ct_right_7_in/1(interp_point_1) -> n-D Lookup Table80/1
  Matrix Multiply72/1 -> Add6/1, Cross Product2/2
  Matrix Multiply76/1 -> Add6/5, Cross Product5/2
  L5/1 -> Out4/1
  Ct_tail_right/3(interp_point_3) -> n-D Lookup Table73/3
  Matrix Multiply74/1 -> Add6/3, Cross Product3/2
  Ct_left_out/2(interp_point_2) -> n-D Lookup Table74/2
  MATLAB Function81/1(Ct_Scale_2) -> Product77/2
  n-D Lookup Table76/1 -> Mux81/1
  Ct_right_7_in/2(interp_point_2) -> n-D Lookup Table80/2
  Matrix Multiply92/1 -> Add6/13, Cross Product13/2
  Ct_left_5/3(interp_point_3) -> n-D Lookup Table78/3
  n-D Lookup Table82/1 -> Mux76/1
  Ct_left_6_in/1(interp_point_1) -> n-D Lookup Table79/1
  Constant100/1 -> Mux75/2
  MATLAB Function85/1(Ct_Scale_6) -> Product81/2
  n-D Lookup Table75/1 -> Mux80/1
  MATLAB Function82/1(Ct_Scale_3) -> Product78/2
  Ct_left_3/1(interp_point_1) -> n-D Lookup Table76/1
  Cross Product13/1 -> Add17/13
  Matrix Multiply73/1 -> Add6/2, Cross Product1/2
  Mux84/1 -> Product83/1
  Constant111/1 -> Mux86/2
  Constant110/1 -> Mux84/2
  MATLAB Function190/1(Wing_Transform) -> Matrix Multiply92/1
  Mux78/1 -> Product77/1
  Ct_left_2/3(interp_point_3) -> n-D Lookup Table75/3
  n-D Lookup Table74/1 -> Mux79/1
  Ct_tail_right/2(interp_point_2) -> n-D Lookup Table73/2
  Constant128/1 -> Cross Product4/1
  Ct_left_2/2(interp_point_2) -> n-D Lookup Table75/2
  Ct_left_6_in/2(interp_point_2) -> n-D Lookup Table79/2
  Product91/1 -> Matrix Multiply91/2
  Matrix Multiply78/1 -> Add6/7, Cross Product7/2
  MATLAB Function187/1(Wing_Transform) -> Matrix Multiply89/1
  Mux87/1 -> Product93/1
  Constant107/1 -> Mux81/2
  n-D Lookup Table72/1 -> Mux74/1
  Constant99/1 -> Mux85/2
  Matrix Multiply77/1 -> Add6/6, Cross Product6/2
  Constant101/1 -> Mux76/2
  MATLAB Function184/1(Wing_Transform) -> Matrix Multiply78/1
  n-D Lookup Table81/1 -> Mux75/1
  Constant103/1 -> Mux74/2
  Product80/1 -> Matrix Multiply76/2
  Constant1/1 -> Cross Product1/1
  Ct_right_9/2(interp_point_2) -> n-D Lookup Table82/2
  Cross Product10/1 -> Add17/10
  Ct_left_4/4(interp_point_4) -> n-D Lookup Table77/4
  MATLAB Function92/1(Ct_Scale_13) -> Product92/2
  Cross Product6/1 -> Add17/6
  Constant138/1 -> Cross Product14/1
  M5/1 -> Out5/1
  Ct_tail_left/3(interp_point_3) -> n-D Lookup Table72/3
  Ct_right_11/2(interp_point_2) -> n-D Lookup Table84/2
  Ct_left_6_in/3(interp_point_3) -> n-D Lookup Table79/3
  Product77/1 -> Matrix Multiply73/2
  Ct_left_5/4(interp_point_4) -> n-D Lookup Table78/4
  Cross Product8/1 -> Add17/8
  Fy4/1 -> Out2/1
  MATLAB Function181/1(Wing_Transform) -> Matrix Multiply75/1
  Product78/1 -> Matrix Multiply74/2
  Ct_tail_right/4(interp_point_4) -> n-D Lookup Table73/4
  Product79/1 -> Matrix Multiply75/2
  Constant137/1 -> Cross Product13/1
  Ct_left_5/2(interp_point_2) -> n-D Lookup Table78/2
  Ct_left_5/1(interp_point_1) -> n-D Lookup Table78/1
  Constant126/1 -> Cross Product2/1
  Product81/1 -> Matrix Multiply77/2
  Ct_tail_left/4(interp_point_4) -> n-D Lookup Table72/4
  n-D Lookup Table84/1 -> Mux86/1
  Product92/1 -> Matrix Multiply92/2
  Ct_left_3/2(interp_point_2) -> n-D Lookup Table76/2
  Matrix Multiply88/1 -> Add6/9, Cross Product9/2
  Constant133/1 -> Cross Product9/1
  Constant106/1 -> Mux80/2
  Constant131/1 -> Cross Product7/1
  Matrix Multiply79/1 -> Add6/8, Cross Product8/2
  Constant104/1 -> Mux78/2
  Constant136/1 -> Cross Product12/1
  Ct_right_8/2(interp_point_2) -> n-D Lookup Table81/2
  Mux79/1 -> Product78/1
  Matrix Multiply93/1 -> Add6/14, Cross Product14/2
  Cross Product1/1 -> Add17/2
  Cross Product4/1 -> Add17/4
  Cross Product9/1 -> Add17/9
  Cross Product14/1 -> Add17/14
  Cross Product3/1 -> Add17/3
  Ct_left_2/4(interp_point_4) -> n-D Lookup Table75/4
  Ct_left_out/3(interp_point_3) -> n-D Lookup Table74/3
  Ct_left_3/3(interp_point_3) -> n-D Lookup Table76/3
  Ct_left_3/4(interp_point_4) -> n-D Lookup Table76/4
  Mux86/1 -> Product92/1
  Ct_left_4/2(interp_point_2) -> n-D Lookup Table77/2
  Ct_left_4/1(interp_point_1) -> n-D Lookup Table77/1
  Ct_left_6_in/4(interp_point_4) -> n-D Lookup Table79/4
  Ct_tail_right/1(interp_point_1) -> n-D Lookup Table73/1
  Mux81/1 -> Product80/1
  Ct_right_7_in/3(interp_point_3) -> n-D Lookup Table80/3
  MATLAB Function189/1(Wing_Transform) -> Matrix Multiply91/1
  MATLAB Function93/1(Ct_Scale_14) -> Product93/2
  Ct_right_8/1(interp_point_1) -> n-D Lookup Table81/1
  Ct_right_7_in/4(interp_point_4) -> n-D Lookup Table80/4
  Ct_right_11/1(interp_point_1) -> n-D Lookup Table84/1
  Mux75/1 -> Product89/1
  MATLAB Function182/1(Wing_Transform) -> Matrix Multiply76/1
  Ct_right_12_out/1(interp_point_1) -> n-D Lookup Table85/1
  Ct_right_8/3(interp_point_3) -> n-D Lookup Table81/3
  Ct_right_11/3(interp_point_3) -> n-D Lookup Table84/3
  Ct_right_12_out/2(interp_point_2) -> n-D Lookup Table85/2
  Cross Product11/1 -> Add17/11
  Cross Product2/1 -> Add17/1
  Ct_right_11/4(interp_point_4) -> n-D Lookup Table84/4
  MATLAB Function178/1(Tail_Transform) -> Matrix Multiply72/1
  Constant129/1 -> Cross Product5/1
  MATLAB Function180/1(Wing_Transform) -> Matrix Multiply74/1
  MATLAB Function186/1(Wing_Transform) -> Matrix Multiply88/1
  Ct_right_9/4(interp_point_4) -> n-D Lookup Table82/4
  MATLAB Function188/1(Wing_Transform) -> Matrix Multiply90/1
  Ct_right_12_out/4(interp_point_4) -> n-D Lookup Table85/4
  MATLAB Function185/1(Wing_Transform) -> Matrix Multiply79/1
  n-D Lookup Table85/1 -> Mux87/1
  MATLAB Function179/1(Tail_Transform) -> Matrix Multiply73/1
  Cross Product12/1 -> Add17/12
  MATLAB Function88/1(Ct_Scale_9) -> Product88/2
  Ct_left_2/1(interp_point_1) -> n-D Lookup Table75/1
  Ct_left_4/3(interp_point_3) -> n-D Lookup Table77/3
  n-D Lookup Table83/1 -> Mux77/1
  MATLAB Function191/1(Wing_Transform) -> Matrix Multiply93/1
  Constant105/1 -> Mux79/2
  MATLAB Function84/1(Ct_Scale_5) -> Product80/2
  MATLAB Function87/1(Ct_Scale_8) -> Product83/2
  Ct_right_9/3(interp_point_3) -> n-D Lookup Table82/3
  Fz4/1 -> Out3/1
  Fx4/1 -> Out1/1
  u19/1 -> MATLAB Function86/1(u), MATLAB Function185/1(u), Ct_left_6_in/1(u), MATLAB Function87/1(u), MATLAB Function186/1(u), Ct_right_7_in/1(u), MATLAB Function88/1(u), MATLAB Function187/1(u), Ct_right_8/1(u), MATLAB Function89/1(u), MATLAB Function188/1(u), Ct_right_9/1(u), MATLAB Function90/1(u), MATLAB Function189/1(u), Ct_right_10/1(u), MATLAB Function91/1(u), MATLAB Function190/1(u), Ct_right_11/1(u), MATLAB Function92/1(u), MATLAB Function191/1(u), Ct_right_12_out/1(u), MATLAB Function93/1(u), MATLAB Function184/1(u), MATLAB Function85/1(u), Ct_left_4/1(u), MATLAB Function183/1(u), MATLAB Function84/1(u), Ct_left_3/1(u), MATLAB Function182/1(u), MATLAB Function83/1(u), Ct_left_2/1(u), MATLAB Function181/1(u), MATLAB Function82/1(u), Ct_left_out/1(u), MATLAB Function180/1(u), MATLAB Function81/1(u), Ct_tail_right/1(u), MATLAB Function179/1(u), MATLAB Function80/1(u), Ct_tail_left/1(u), MATLAB Function178/1(u), Ct_left_5/1(u)
